simulink model "Sensors_UltraStick25e"  (R2016b)
settings: Solver=VariableStepAuto  StartTime=0.0  StopTime=10.0  RelTol=1e-3
libraries: Sensors_Lib x11
settings Model: Creator=UAVLAB  LastModifiedBy=hollysfolders

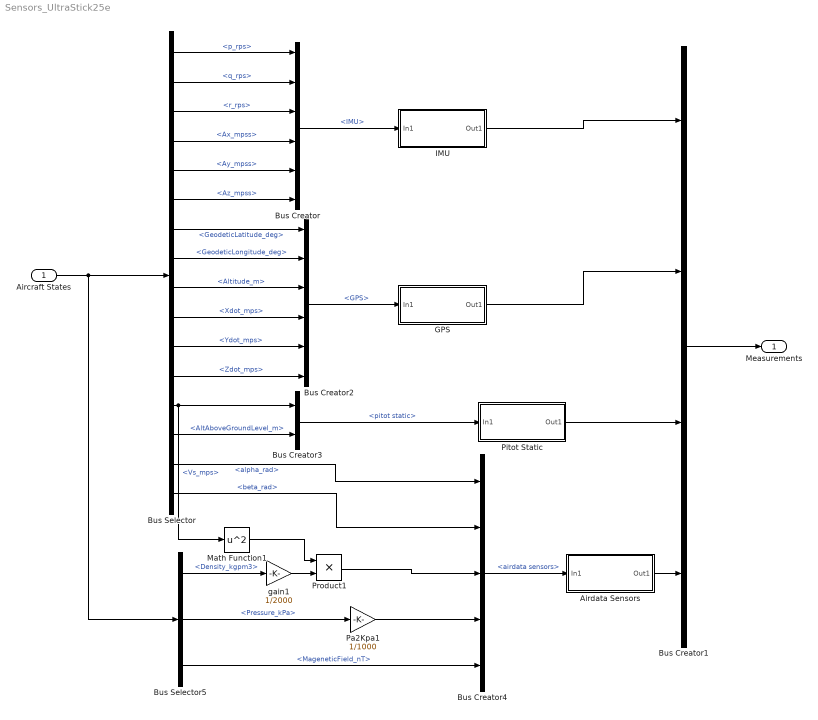
== system Sensors_UltraStick25e ==
  Aircraft States : Inport  OutDataTypeStr=Bus: States
  Airdata Sensors : Subsystem
  Bus Creator : BusCreator  Inputs=6
  Bus Creator1 : BusCreator  Inputs=4  OutDataTypeStr=Bus: Sensors
      settings: InheritFromInputs=off
  Bus Creator2 : BusCreator  Inputs=6
  Bus Creator3 : BusCreator  Inputs=2
  Bus Creator4 : BusCreator  Inputs=5
  Bus Selector : BusSelector  OutputSignals=RigidStates.AngVel.p_rps,RigidStates.AngVel.q_rps,RigidStates.AngVel.r_rps,RigidStates.Accels.Ax_mpss,RigidStates.Accels.Ay_mpss,RigidStates.Accels.Az_mpss,AuxVar.Nav.GeodeticLatitude_deg,AuxVar.Nav.GeodeticLongitude_deg,AuxVar.Nav.Altitude_m,AuxVar.V_e.Xdot_mps,AuxVar.V_e.Ydot_mps,AuxVar.V_e.Zdot_mps,AuxVar.WindAxesParams.Vs_mps,AuxVar.Nav.AltAboveGroundLevel_m,AuxVar.WindAxesParams.alpha_rad,AuxVar.WindAxesParams.beta_rad
  Bus Selector5 : BusSelector  OutputSignals=EnvData.Density_kgpm3,EnvData.Pressure_kPa,EnvData.MageneticField_nT
  GPS : Subsystem
  IMU : Subsystem
  Math Function1 : Math  Operator=square  SaturateOnIntegerOverflow=on
  Pa2Kpa1 : Gain  Gain=1/1000
  Pitot Static : Subsystem
  Product1 : Product  RndMeth=Zero
  gain1 : Gain  Gain=1/2000
  Measurements : Outport  OutDataTypeStr=Bus: Sensors
  wires:
  Aircraft States/1 -> Bus Selector/1, Bus Selector5/1
  Bus Creator1/1 -> Measurements/1
  Bus Selector/1 -> Bus Creator/1  "<p_rps>"
  Bus Selector/2 -> Bus Creator/2  "<q_rps>"
  Bus Selector/3 -> Bus Creator/3  "<r_rps>"
  Bus Selector/4 -> Bus Creator/4  "<Ax_mpss>"
  Bus Selector/5 -> Bus Creator/5  "<Ay_mpss>"
  Bus Selector/6 -> Bus Creator/6  "<Az_mpss>"
  Bus Selector/8 -> Bus Creator2/2  "<GeodeticLongitude_deg>"
  Bus Selector/14 -> Bus Creator3/2  "<AltAboveGroundLevel_m>"
  Bus Selector/15 -> Bus Creator4/1  "<alpha_rad>"
  Bus Selector/16 -> Bus Creator4/2  "<beta_rad>"
  Bus Selector/7 -> Bus Creator2/1  "<GeodeticLatitude_deg>"
  Bus Selector/9 -> Bus Creator2/3  "<Altitude_m>"
  Bus Selector/10 -> Bus Creator2/4  "<Xdot_mps>"
  Bus Selector/11 -> Bus Creator2/5  "<Ydot_mps>"
  Bus Selector/12 -> Bus Creator2/6  "<Zdot_mps>"
  Bus Selector/13 -> Math Function1/1, Bus Creator3/1  "<Vs_mps>"
  Product1/1 -> Bus Creator4/3
  gain1/1 -> Product1/2
  Math Function1/1 -> Product1/1
  Bus Selector5/1 -> gain1/1  "<Density_kgpm3>"
  Pa2Kpa1/1 -> Bus Creator4/4
  Bus Selector5/2 -> Pa2Kpa1/1  "<Pressure_kPa>"
  Bus Selector5/3 -> Bus Creator4/5  "<MageneticField_nT>"
  Bus Creator/1 -> IMU/1(In1)  "<IMU>"
  Bus Creator2/1 -> GPS/1(In1)  "<GPS>"
  Bus Creator3/1 -> Pitot Static/1(In1)  "<pitot static>"
  Bus Creator4/1 -> Airdata Sensors/1(In1)  "<airdata sensors>"
  IMU/1(Out1) -> Bus Creator1/1
  GPS/1(Out1) -> Bus Creator1/2
  Pitot Static/1(Out1) -> Bus Creator1/3
  Airdata Sensors/1(Out1) -> Bus Creator1/4

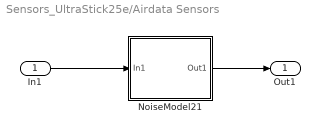
== system Sensors_UltraStick25e/Airdata Sensors ==
  In1 : Inport
  NoiseModel21 : Subsystem  Variant=on  VariantControl=Variant1
  Out1 : Outport
  wires:
  In1/1 -> NoiseModel21/1("In1 ")
  NoiseModel21/1(" Out1") -> Out1/1

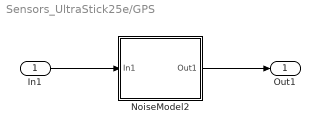
== system Sensors_UltraStick25e/GPS ==
  In1 : Inport
  NoiseModel2 : Subsystem  Variant=on  VariantControl=AC_IMU_TYPE1
  Out1 : Outport
  wires:
  In1/1 -> NoiseModel2/1("In1 ")
  NoiseModel2/1(" Out1") -> Out1/1

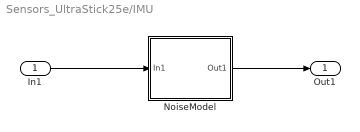
== system Sensors_UltraStick25e/IMU ==
  In1 : Inport
  NoiseModel : Subsystem  Variant=on  VariantControl=Variant1
  Out1 : Outport
  wires:
  In1/1 -> NoiseModel/1("In1 ")
  NoiseModel/1(" Out1") -> Out1/1

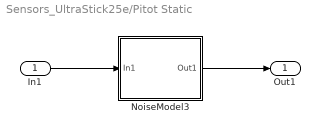
== system Sensors_UltraStick25e/Pitot Static ==
  In1 : Inport
  NoiseModel3 : Subsystem  Variant=on  VariantControl=Variant1
  Out1 : Outport
  wires:
  In1/1 -> NoiseModel3/1("In1 ")
  NoiseModel3/1(" Out1") -> Out1/1

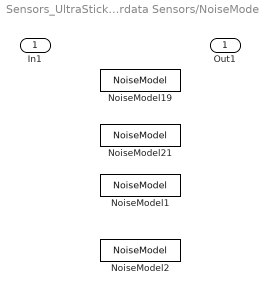
== system Sensors_UltraStick25e/Airdata Sensors/NoiseModel21 ==
  "In1 " : Inport
  NoiseModel1 : Sensors_Lib/NoiseModel  VariantControl=AC_AIRDATA_TYPE3  noise_on=AC.Sensors.NoiseOn  sigma=AC.Sensors.AirData.alpha_noise  seed=87828  bias=AC.Sensors.AirData.alpha_bias  scf=AC.Sensors.AirData.alpha_scf  timestep=SampleTime
  NoiseModel19 : Sensors_Lib/NoiseModel  VariantControl=AC_AIRDATA_TYPE1  noise_on=AC.Sensors.NoiseOn  sigma=AC.Sensors.AirData.beta_noise  seed=87828  bias=AC.Sensors.AirData.beta_bias  scf=AC.Sensors.AirData.beta_scf  timestep=SampleTime
  NoiseModel2 : Sensors_Lib/NoiseModel  VariantControl=AC_AIRDATA_TYPE4  noise_on=AC.Sensors.NoiseOn  sigma=AC.Sensors.AirData.alpha_noise  seed=87828  bias=AC.Sensors.AirData.alpha_bias  scf=AC.Sensors.AirData.alpha_scf  timestep=SampleTime
  NoiseModel21 : Sensors_Lib/NoiseModel  VariantControl=AC_AIRDATA_TYPE2  noise_on=AC.Sensors.NoiseOn  sigma=AC.Sensors.AirData.alpha_noise  seed=87828  bias=AC.Sensors.AirData.alpha_bias  scf=AC.Sensors.AirData.alpha_scf  timestep=SampleTime
  " Out1" : Outport

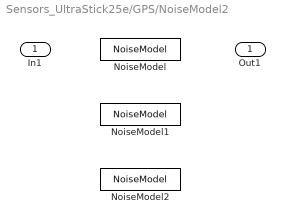
== system Sensors_UltraStick25e/GPS/NoiseModel2 ==
  "In1 " : Inport
  NoiseModel : Sensors_Lib/NoiseModel  VariantControl=AC_GPS_TYPE1  noise_on=AC.Sensors.NoiseOn  sigma=AC.Sensors.IMU.p_noise  seed=878230  bias=AC.Sensors.IMU.p_bias  scf=AC.Sensors.IMU.p_scf  timestep=SampleTime
  NoiseModel1 : Sensors_Lib/NoiseModel  VariantControl=AC_GPS_TYPE2  noise_on=AC.Sensors.NoiseOn  sigma=AC.Sensors.IMU.p_noise  seed=878230  bias=AC.Sensors.IMU.p_bias  scf=AC.Sensors.IMU.p_scf  timestep=SampleTime
  NoiseModel2 : Sensors_Lib/NoiseModel  VariantControl=AC_GPS_TYPE3  noise_on=AC.Sensors.NoiseOn  sigma=AC.Sensors.IMU.p_noise  seed=878230  bias=AC.Sensors.IMU.p_bias  scf=AC.Sensors.IMU.p_scf  timestep=SampleTime
  " Out1" : Outport

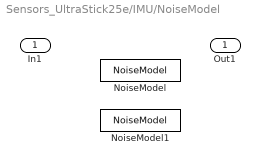
== system Sensors_UltraStick25e/IMU/NoiseModel ==
  "In1 " : Inport
  NoiseModel : Sensors_Lib/NoiseModel  VariantControl=AC_IMU_TYPE1  noise_on=AC.Sensors.NoiseOn  sigma=AC.Sensors.IMU.p_noise  seed=878230  bias=AC.Sensors.IMU.p_bias  scf=AC.Sensors.IMU.p_scf  timestep=SampleTime
  NoiseModel1 : Sensors_Lib/NoiseModel  VariantControl=AC_IMU_TYPE2  noise_on=AC.Sensors.NoiseOn  sigma=AC.Sensors.IMU.p_noise  seed=878230  bias=AC.Sensors.IMU.p_bias  scf=AC.Sensors.IMU.p_scf  timestep=SampleTime
  " Out1" : Outport

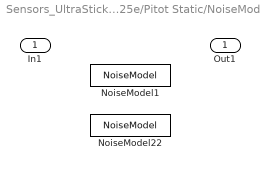
== system Sensors_UltraStick25e/Pitot Static/NoiseModel3 ==
  "In1 " : Inport
  NoiseModel1 : Sensors_Lib/NoiseModel  VariantControl=AC_PITOT_TYPE1  noise_on=AC.Sensors.NoiseOn  sigma=AC.Sensors.AirData.ias_noise  seed=878236  bias=AC.Sensors.AirData.ias_bias  scf=AC.Sensors.AirData.ias_scf  timestep=SampleTime
  NoiseModel22 : Sensors_Lib/NoiseModel  VariantControl=AC_PITOT_TYPE2  noise_on=AC.Sensors.NoiseOn  sigma=AC.Sensors.AirData.ias_noise  seed=878236  bias=AC.Sensors.AirData.ias_bias  scf=AC.Sensors.AirData.ias_scf  timestep=SampleTime
  " Out1" : Outport
